simulink model "twelveBalls"  (R2024a)
settings: Solver=FixedStepAuto  StartTime=0.0  StopTime=config.t_max  FixedStep=config.timestep  RelTol=1e-3
undefined symbols (not defined in the file or in its folder): agentsInfo, config, DiscIntNeverNeededParam, Sim3dSensor
libraries: sim3dlib x14, dspvision x1, visionsinks x1
(part 1 of 2)
settings Model: Creator=alexs  LastModifiedBy=alexs

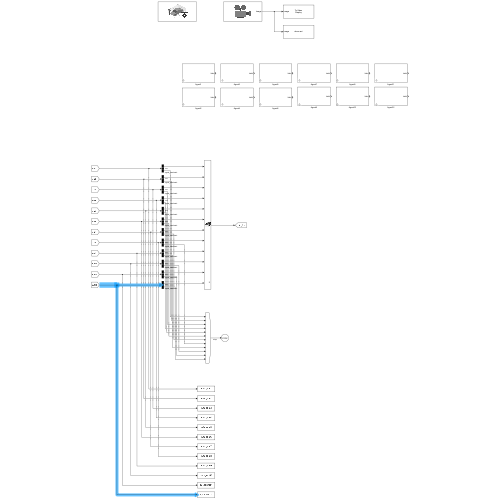
[thumbnail: Simulink's stored preview of the top-level diagram]
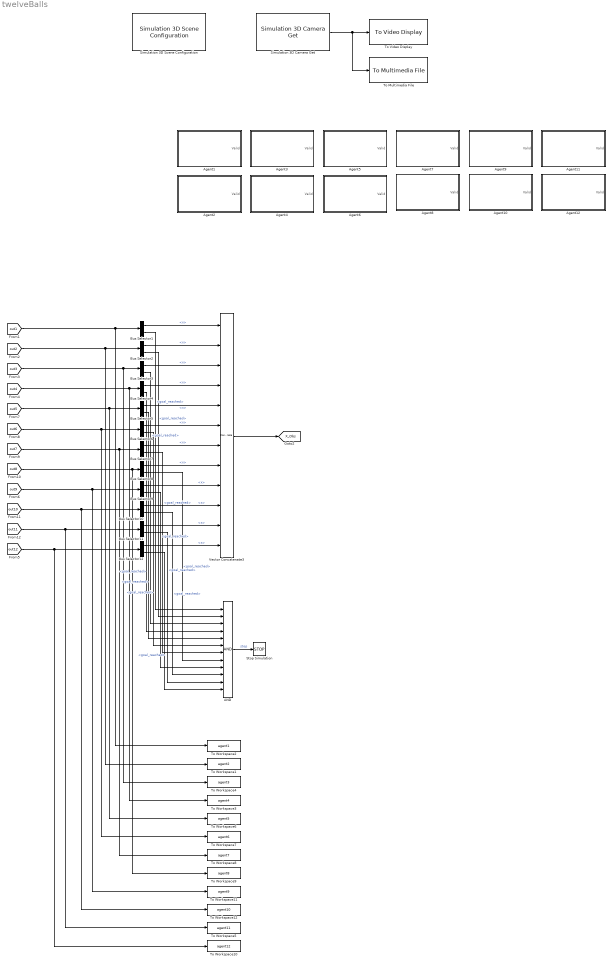
== system twelveBalls ==
  AND : Logic  Inputs=12  IconShape=distinctive  AllPortsSameDT=off  OutDataTypeStr=boolean
  Agent1 : Subsystem  mask{id=1, allAgentsInfo=agentsInfo}
      mask prompts: id "Identifier"; allAgentsInfo "Agents information"
  Agent10 : Subsystem  mask{id=10, allAgentsInfo=agentsInfo}
      mask prompts: id "Identifier"; allAgentsInfo "Agents information"
  Agent11 : Subsystem  mask{id=11, allAgentsInfo=agentsInfo}
      mask prompts: id "Identifier"; allAgentsInfo "Agents information"
  Agent12 : Subsystem  mask{id=12, allAgentsInfo=agentsInfo}
      mask prompts: id "Identifier"; allAgentsInfo "Agents information"
  Agent2 : Subsystem  mask{id=2, allAgentsInfo=agentsInfo}
      mask prompts: id "Identifier"; allAgentsInfo "Agents information"
  Agent3 : Subsystem  mask{id=3, allAgentsInfo=agentsInfo}
      mask prompts: id "Identifier"; allAgentsInfo "Agents information"
  Agent4 : Subsystem  mask{id=4, allAgentsInfo=agentsInfo}
      mask prompts: id "Identifier"; allAgentsInfo "Agents information"
  Agent5 : Subsystem  mask{id=5, allAgentsInfo=agentsInfo}
      mask prompts: id "Identifier"; allAgentsInfo "Agents information"
  Agent6 : Subsystem  mask{id=6, allAgentsInfo=agentsInfo}
      mask prompts: id "Identifier"; allAgentsInfo "Agents information"
  Agent7 : Subsystem  mask{id=7, allAgentsInfo=agentsInfo}
      mask prompts: id "Identifier"; allAgentsInfo "Agents information"
  Agent8 : Subsystem  mask{id=8, allAgentsInfo=agentsInfo}
      mask prompts: id "Identifier"; allAgentsInfo "Agents information"
  Agent9 : Subsystem  mask{id=9, allAgentsInfo=agentsInfo}
      mask prompts: id "Identifier"; allAgentsInfo "Agents information"
  Bus Selector{1..12} (12 alike) : BusSelector  OutputSignals=x,goal_reached
  Simulation 3D Camera Get : sim3dlib/Simulation 3D Camera Get  Priority=1  sensorTag=Sim3dSensor�  sensorId=1  sensorName=Sim3dSensor�  vehTagList={'Scene Origin';'actor1'}  vehTag=Scene Origin  mountLoc=Origin  offsetFlag=on  tmountOffset=cameraTranslation  rmountOffset=cameraRotation  HorizontalResolution=1280  VerticalResolution=720  HorizontalFOV=60  SampleTime=-1  mountPoint=[0 0 20]  mountOrientation=[0 -90 -90]  aMode=5  ID=1
      settings: LibrarySourceBlock=sl3dlib/Simulation 3D/Utilities/Simulation 3D Camera Get
  Simulation 3D Scene Configuration : sim3dlib/Simulation 3D Scene Configuration  Priority=0  ProjectFormat=Default Scenes  SceneDesc=Empty scene  ProjectName=C:\Program Files\MATLAB\R2024a\toolbox\shared\sim3d_projects\automotive_project_windows\UE\WindowsNoEditor\VehicleSimulation.exe  ScenePath=/Game/Maps/HwStrght  EnableOpenDRIVE=off  vehTagList={'Custom';'Scene Origin'}  vehTag=Scene Origin  FreeCameraInitialTranslation=[0, 0, 0]  FreeCameraDefaultInitialTranslation=[-6, 0, 2]  FreeCameraInitialRotation=[0, 0, 0]  FreeCameraDefaultInitialRotation=[0, -15, 0]  OpVisEn=off  Ts=config.timestep  EnableWindow=off  EnableRemoteAccess=off  EnableWeather=off  SunAzimuth=90  SunAltitude=40.0  EnableGeospatialSun=off  Latitude=0  Longitude=0  Date=2023-01-01  Time=10:30:00  GeoTimeZone=-5.0  SunDaylightSaving=off  wind=1  clouds=10  EnableVolumetricClouds=off  CloudCoverage=0  CloudAltitude=6  fog=0  rain=0  RaindropsEffect=off  SnowDensity=0  EnableGeospatial=off  UseTrueOrigin=off  OriginHeight=200  OriginLatitude=40.744652  OriginLongitude=-73.988864  MapStyle=Aerial  AdditionalAssetIDs=[]  UseAdvancedSunSky=off  SolarTime=11  TimeZone=-5  Day=21  Month=9  Year=2022  UseDaylightSavingTime=on  DSTStartDay=10  DSTStartMonth=3  DSTEndDay=3  DSTEndMonth=11  DSTSwitchHour=2  sensorTag=MainCamera1  sensorId=1  sensorName=MainCamera1  mountLoc=Origin  offsetFlag=off  tmountOffset=[0, 0, 0]  rmountOffset=[0, 0, 0]  HorizontalResolution=1280  VerticalResolution=720  HorizontalFOV=60  mountPoint=[0 0 0]  mountOrientation=[0 0 0]  aMode=5  ID=1  GeoTrigger=Inactive
      settings: LibrarySourceBlock=sl3dlib/Simulation 3D/Environment/Simulation 3D Scene Configuration
  Stop Simulation : Stop
  To Multimedia File : dspvision/To Multimedia File  outputFilename=demo.avi  streamSelection=Video only  videoCompressor=None (uncompressed)  audioCompressor=None (uncompressed)  imagePorts=One multidimensional signal  fileType=AVI  audioDatatype=Determine from input data type  fourcc=RGB  audioBitRate=128  audioQuality=75  videoQuality=75  mj2000CompFactor=10
      settings: LibrarySourceBlock=visionsinks/To Multimedia File
  To Video Display : visionsinks/To Video Display  windowSizeMode=Normal  openAtMdlStart=on  fullScreen=off  videoWindowX=678  videoWindowY=374  saveWindowSize=off  videoWindowWidth=1052  videoWindowHeight=706  inputColorFormat=RGB  inputType=Obsolete  imagePorts=One multidimensional signal  OutputDevice=On-screen video monitor  dataOrg=Column-major  isWindowOpen=off
  To Workspace1 : ToWorkspace  VariableName=agent2  SaveFormat=Timeseries  SampleTime=-1
  To Workspace10 : ToWorkspace  VariableName=agent12  SaveFormat=Timeseries  SampleTime=-1
  To Workspace11 : ToWorkspace  VariableName=agent9  SaveFormat=Timeseries  SampleTime=-1
  To Workspace12 : ToWorkspace  VariableName=agent10  SaveFormat=Timeseries  SampleTime=-1
  To Workspace2 : ToWorkspace  VariableName=agent1  SaveFormat=Timeseries  SampleTime=-1
  To Workspace3 : ToWorkspace  VariableName=agent4  SaveFormat=Timeseries  SampleTime=-1
  To Workspace4 : ToWorkspace  VariableName=agent3  SaveFormat=Timeseries  SampleTime=-1
  To Workspace5 : ToWorkspace  VariableName=agent11  SaveFormat=Timeseries  SampleTime=-1
  To Workspace6 : ToWorkspace  VariableName=agent5  SaveFormat=Timeseries  SampleTime=-1
  To Workspace7 : ToWorkspace  VariableName=agent6  SaveFormat=Timeseries  SampleTime=-1
  To Workspace8 : ToWorkspace  VariableName=agent7  SaveFormat=Timeseries  SampleTime=-1
  To Workspace9 : ToWorkspace  VariableName=agent8  SaveFormat=Timeseries  SampleTime=-1
  Vector Concatenate3 : Concatenate  NumInputs=12  Mode=Multidimensional array  ConcatenateDimension=2
  tag scope: X_Obs=global
  wires:
  Simulation 3D Camera Get/1 -> To Multimedia File/1, To Video Display/1
  Bus Selector7/1 -> Vector Concatenate3/7  "<x>"
  Bus Selector3/2 -> AND/3  "<goal_reached>"
  [out1] -> Bus Selector1/1, To Workspace2/1
  Bus Selector1/1 -> Vector Concatenate3/1  "<x>"
  [out7] -> Bus Selector7/1, To Workspace8/1
  [out4] -> Bus Selector4/1, To Workspace3/1
  Bus Selector2/1 -> Vector Concatenate3/2  "<x>"
  Bus Selector8/2 -> AND/8  "<goal_reached>"
  [out2] -> Bus Selector2/1, To Workspace1/1
  Vector Concatenate3/1 -> [X_Obs]
  [out8] -> Bus Selector8/1, To Workspace9/1
  Bus Selector1/2 -> AND/1  "<goal_reached>"
  [out3] -> Bus Selector3/1, To Workspace4/1
  Bus Selector6/2 -> AND/6  "<goal_reached>"
  Bus Selector5/2 -> AND/5  "<goal_reached>"
  Bus Selector2/2 -> AND/2  "<goal_reached>"
  [out6] -> To Workspace7/1, Bus Selector6/1
  Bus Selector4/2 -> AND/4  "<goal_reached>"
  Bus Selector8/1 -> Vector Concatenate3/8  "<x>"
  Bus Selector3/1 -> Vector Concatenate3/3  "<x>"
  Bus Selector4/1 -> Vector Concatenate3/4  "<x>"
  Bus Selector6/1 -> Vector Concatenate3/6  "<x>"
  [out5] -> Bus Selector5/1, To Workspace6/1
  Bus Selector7/2 -> AND/7  "<goal_reached>"
  AND/1 -> Stop Simulation/1  "stop"
  Bus Selector5/1 -> Vector Concatenate3/5  "<x>"
  [out9] -> To Workspace11/1, Bus Selector9/1
  [out10] -> To Workspace12/1, Bus Selector10/1
  [out11] -> To Workspace5/1, Bus Selector11/1
  [out12] -> To Workspace10/1, Bus Selector12/1
  Bus Selector9/1 -> Vector Concatenate3/9  "<x>"
  Bus Selector10/1 -> Vector Concatenate3/10  "<x>"
  Bus Selector11/1 -> Vector Concatenate3/11  "<x>"
  Bus Selector12/1 -> Vector Concatenate3/12  "<x>"
  Bus Selector9/2 -> AND/9  "<goal_reached>"
  Bus Selector10/2 -> AND/10  "<goal_reached>"
  Bus Selector11/2 -> AND/11  "<goal_reached>"
  Bus Selector12/2 -> AND/12  "<goal_reached>"

== system twelveBalls/Agent1 ==
  Actor : Subsystem
  Bus Selector1 : BusSelector  OutputSignals=u
  Controller : Subsystem  mask{id=id, allAgentsInfo=agentsInfo}
      mask prompts: id "Identifier"; allAgentsInfo "Information for all agents"
  Valid : Outport
  tag scope: out1=global
  wires:
  Actor/3(v) -> Controller/2(v)
  Controller/1(out_data) -> Bus Selector1/1, [out1]
  Actor/2(p) -> Controller/1(p)
  Bus Selector1/1 -> Actor/1(u_in)  "<u>"
  [X_Obs] -> Controller/3(X_Obs)
  Actor/1(Valid) -> Valid/1
  Actor/4(overlap_event) -> Controller/4(overlap_event)

== system twelveBalls/Agent10 ==
  Actor : Subsystem
  Bus Selector1 : BusSelector  OutputSignals=u
  Controller : Subsystem  mask{id=id, allAgentsInfo=agentsInfo}
      mask prompts: id "Identifier"; allAgentsInfo "Information for all agents"
  Valid : Outport
  tag scope: out10=global
  wires:
  Actor/3(v) -> Controller/2(v)
  Controller/1(out_data) -> Bus Selector1/1, [out10]
  Actor/2(p) -> Controller/1(p)
  Bus Selector1/1 -> Actor/1(u_in)  "<u>"
  [X_Obs] -> Controller/3(X_Obs)
  Actor/1(Valid) -> Valid/1
  Actor/4(overlap_event) -> Controller/4(overlap_event)

== system twelveBalls/Agent11 ==
  Actor : Subsystem
  Bus Selector1 : BusSelector  OutputSignals=u
  Controller : Subsystem  mask{id=id, allAgentsInfo=agentsInfo}
      mask prompts: id "Identifier"; allAgentsInfo "Information for all agents"
  Valid : Outport
  tag scope: out11=global
  wires:
  Actor/4(overlap_event) -> Controller/4(overlap_event)
  Actor/1(Valid) -> Valid/1
  [X_Obs] -> Controller/3(X_Obs)
  Bus Selector1/1 -> Actor/1(u_in)  "<u>"
  Actor/2(p) -> Controller/1(p)
  Controller/1(out_data) -> [out11], Bus Selector1/1
  Actor/3(v) -> Controller/2(v)

== system twelveBalls/Agent12 ==
  Actor : Subsystem
  Bus Selector1 : BusSelector  OutputSignals=u
  Controller : Subsystem  mask{id=id, allAgentsInfo=agentsInfo}
      mask prompts: id "Identifier"; allAgentsInfo "Information for all agents"
  Valid : Outport
  tag scope: out12=global
  wires:
  Actor/3(v) -> Controller/2(v)
  Controller/1(out_data) -> Bus Selector1/1, [out12]
  Actor/2(p) -> Controller/1(p)
  Bus Selector1/1 -> Actor/1(u_in)  "<u>"
  [X_Obs] -> Controller/3(X_Obs)
  Actor/1(Valid) -> Valid/1
  Actor/4(overlap_event) -> Controller/4(overlap_event)

== system twelveBalls/Agent2 ==
  Actor : Subsystem
  Bus Selector1 : BusSelector  OutputSignals=u
  Controller : Subsystem  mask{id=id, allAgentsInfo=agentsInfo}
      mask prompts: id "Identifier"; allAgentsInfo "Information for all agents"
  Valid : Outport
  tag scope: out2=global
  wires:
  Actor/4(overlap_event) -> Controller/4(overlap_event)
  Actor/1(Valid) -> Valid/1
  [X_Obs] -> Controller/3(X_Obs)
  Bus Selector1/1 -> Actor/1(u_in)  "<u>"
  Actor/2(p) -> Controller/1(p)
  Controller/1(out_data) -> [out2], Bus Selector1/1
  Actor/3(v) -> Controller/2(v)

== system twelveBalls/Agent3 ==
  Actor : Subsystem
  Bus Selector1 : BusSelector  OutputSignals=u
  Controller : Subsystem  mask{id=id, allAgentsInfo=agentsInfo}
      mask prompts: id "Identifier"; allAgentsInfo "Information for all agents"
  Valid : Outport
  tag scope: out3=global
  wires:
  Actor/3(v) -> Controller/2(v)
  Controller/1(out_data) -> Bus Selector1/1, [out3]
  Actor/2(p) -> Controller/1(p)
  Bus Selector1/1 -> Actor/1(u_in)  "<u>"
  [X_Obs] -> Controller/3(X_Obs)
  Actor/1(Valid) -> Valid/1
  Actor/4(overlap_event) -> Controller/4(overlap_event)

== system twelveBalls/Agent4 ==
  Actor : Subsystem
  Bus Selector1 : BusSelector  OutputSignals=u
  Controller : Subsystem  mask{id=id, allAgentsInfo=agentsInfo}
      mask prompts: id "Identifier"; allAgentsInfo "Information for all agents"
  Valid : Outport
  tag scope: out4=global
  wires:
  Actor/4(overlap_event) -> Controller/4(overlap_event)
  Actor/1(Valid) -> Valid/1
  [X_Obs] -> Controller/3(X_Obs)
  Bus Selector1/1 -> Actor/1(u_in)  "<u>"
  Actor/2(p) -> Controller/1(p)
  Controller/1(out_data) -> [out4], Bus Selector1/1
  Actor/3(v) -> Controller/2(v)

== system twelveBalls/Agent5 ==
  Actor : Subsystem
  Bus Selector1 : BusSelector  OutputSignals=u
  Controller : Subsystem  mask{id=id, allAgentsInfo=agentsInfo}
      mask prompts: id "Identifier"; allAgentsInfo "Information for all agents"
  Valid : Outport
  tag scope: out5=global
  wires:
  Actor/4(overlap_event) -> Controller/4(overlap_event)
  Actor/1(Valid) -> Valid/1
  [X_Obs] -> Controller/3(X_Obs)
  Bus Selector1/1 -> Actor/1(u_in)  "<u>"
  Actor/2(p) -> Controller/1(p)
  Controller/1(out_data) -> [out5], Bus Selector1/1
  Actor/3(v) -> Controller/2(v)

== system twelveBalls/Agent6 ==
  Actor : Subsystem
  Bus Selector1 : BusSelector  OutputSignals=u
  Controller : Subsystem  mask{id=id, allAgentsInfo=agentsInfo}
      mask prompts: id "Identifier"; allAgentsInfo "Information for all agents"
  Valid : Outport
  tag scope: out6=global
  wires:
  Actor/3(v) -> Controller/2(v)
  Controller/1(out_data) -> Bus Selector1/1, [out6]
  Actor/2(p) -> Controller/1(p)
  Bus Selector1/1 -> Actor/1(u_in)  "<u>"
  [X_Obs] -> Controller/3(X_Obs)
  Actor/1(Valid) -> Valid/1
  Actor/4(overlap_event) -> Controller/4(overlap_event)

== system twelveBalls/Agent7 ==
  Actor : Subsystem
  Bus Selector1 : BusSelector  OutputSignals=u
  Controller : Subsystem  mask{id=id, allAgentsInfo=agentsInfo}
      mask prompts: id "Identifier"; allAgentsInfo "Information for all agents"
  Valid : Outport
  tag scope: out7=global
  wires:
  Actor/3(v) -> Controller/2(v)
  Controller/1(out_data) -> Bus Selector1/1, [out7]
  Actor/2(p) -> Controller/1(p)
  Bus Selector1/1 -> Actor/1(u_in)  "<u>"
  [X_Obs] -> Controller/3(X_Obs)
  Actor/1(Valid) -> Valid/1
  Actor/4(overlap_event) -> Controller/4(overlap_event)

== system twelveBalls/Agent8 ==
  Actor : Subsystem
  Bus Selector1 : BusSelector  OutputSignals=u
  Controller : Subsystem  mask{id=id, allAgentsInfo=agentsInfo}
      mask prompts: id "Identifier"; allAgentsInfo "Information for all agents"
  Valid : Outport
  tag scope: out8=global
  wires:
  Actor/4(overlap_event) -> Controller/4(overlap_event)
  Actor/1(Valid) -> Valid/1
  [X_Obs] -> Controller/3(X_Obs)
  Bus Selector1/1 -> Actor/1(u_in)  "<u>"
  Actor/2(p) -> Controller/1(p)
  Controller/1(out_data) -> [out8], Bus Selector1/1
  Actor/3(v) -> Controller/2(v)

== system twelveBalls/Agent9 ==
  Actor : Subsystem
  Bus Selector1 : BusSelector  OutputSignals=u
  Controller : Subsystem  mask{id=id, allAgentsInfo=agentsInfo}
      mask prompts: id "Identifier"; allAgentsInfo "Information for all agents"
  Valid : Outport
  tag scope: out9=global
  wires:
  Actor/4(overlap_event) -> Controller/4(overlap_event)
  Actor/1(Valid) -> Valid/1
  [X_Obs] -> Controller/3(X_Obs)
  Bus Selector1/1 -> Actor/1(u_in)  "<u>"
  Actor/2(p) -> Controller/1(p)
  Controller/1(out_data) -> [out9], Bus Selector1/1
  Actor/3(v) -> Controller/2(v)

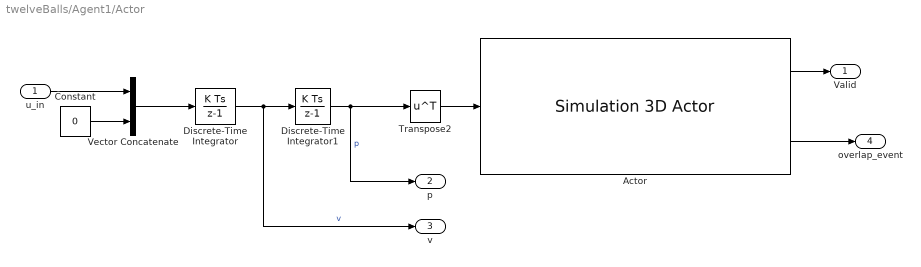
== system twelveBalls/Agent1/Actor ==
  u_in : Inport
  Actor : sim3dlib/Simulation 3D Actor  Priority=1  ActorName=actor1  ParentName=Scene Origin  Operation=Create at setup  InitScriptText=|  SampleTime=-1  Translation=agentsInfo{id}.p'  Rotation=single([0 0 0])  Scale=single([1 1 1])  InputsText=actor1.Translation  EventsText=actor1.BeginOverlapEvent  aMode=5  ActorTag=actor1  ActorType=Sim3dActor  ID=C
      | % Reserved keywords:
      | % - Actor : handle to this actor object
      | % - World : handle to the world object
      | 
      | % Examples:
      | 
      | % Create a primitive geometry (optional)
      | 
      | % Actor.createShape('sphere', [allAgentsInfo{id}.shape(1) allAgentsInfo{id}.shape(2) 1]);
      | 
      | 
      | % Initialize values (optional)
      | % Actor.Scale = 1;
      | % Actor.Gravity = false;
      | % Actor.Physics = true;
      | % Actor.Color = [0 0 1];
      | % Actor.Shininess = 0;
      | % Actor.Mobility = sim3d.utils.MobilityTypes.Movable;
      | % Actor.Shadows = false;
  Constant : Constant  Value=0
  Discrete-Time Integrator : DiscreteIntegrator  InitialCondition=agentsInfo{id}.v  SampleTime=-1  LimitOutput=on  UpperSaturationLimit=config.v_max/sqrt(2)  LowerSaturationLimit=-config.v_max/sqrt(2)  ICPrevOutput=DiscIntNeverNeededParam  ICPrevScaledInput=DiscIntNeverNeededParam
  Discrete-Time Integrator1 : DiscreteIntegrator  InitialCondition=agentsInfo{id}.p  SampleTime=-1  ICPrevOutput=DiscIntNeverNeededParam  ICPrevScaledInput=DiscIntNeverNeededParam
  Transpose2 : Math  Operator=transpose
  Vector Concatenate : Concatenate
  Valid : Outport
  p : Outport  Port=2
  v : Outport  Port=3
  overlap_event : Outport  Port=4
  wires:
  Actor/1 -> Valid/1
  Discrete-Time Integrator1/1 -> Transpose2/1, p/1  "p"
  Discrete-Time Integrator/1 -> Discrete-Time Integrator1/1, v/1  "v"
  Transpose2/1 -> Actor/1
  u_in/1 -> Vector Concatenate/1
  Constant/1 -> Vector Concatenate/2
  Vector Concatenate/1 -> Discrete-Time Integrator/1
  Actor/2 -> overlap_event/1

== system twelveBalls/Agent1/Controller ==
  p : Inport
  v : Inport  Port=2
  X_Obs : Inport  Port=3
  overlap_event : Inport  Port=4
  Bus Creator : BusCreator  Inputs=6
  Clock1 : Clock
  Stop Simulation : Stop
  Vector Concatenate2 : Concatenate
  h_cbf : MATLABSystem  System=h_cbf_system  id=id  config=config  agents_info=agentsInfo  SimulateUsing=Interpreted execution
      mask Type: h_cbf_system
      mask Display:
      | disp('h_cbf_system');
      | port_label('input',1,'t');
      | port_label('input',2,'x');
      | port_label('input',3,'X_obs');
      | port_label('output',1,'u');
      | port_label('output',2,'goal_reached');
      | port_label('output',3,'cost');
      | port_label('output',4,'exit_flag');
  out_data : Outport
  wires:
  Vector Concatenate2/1 -> h_cbf/2, Bus Creator/5  "x"
  h_cbf/4 -> Stop Simulation/1, Bus Creator/4  "exit_flag"
  Bus Creator/1 -> out_data/1
  Clock1/1 -> h_cbf/1
  h_cbf/3 -> Bus Creator/3  "cost"
  p/1 -> Vector Concatenate2/1
  h_cbf/1 -> Bus Creator/1  "u"
  v/1 -> Vector Concatenate2/2
  X_Obs/1 -> h_cbf/3
  h_cbf/2 -> Bus Creator/2  "goal_reached"
  overlap_event/1 -> Bus Creator/6  "overlap_event"

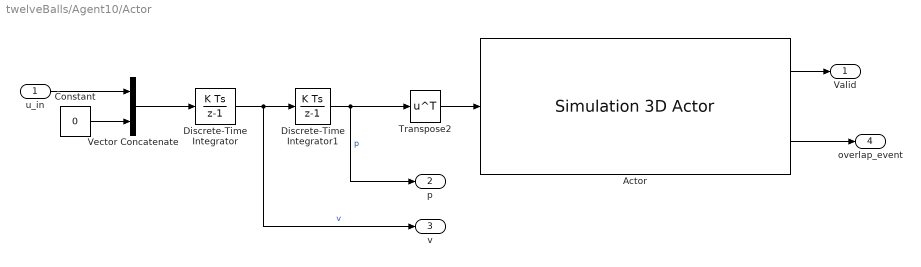
== system twelveBalls/Agent10/Actor ==
  u_in : Inport
  Actor : sim3dlib/Simulation 3D Actor  Priority=1  ActorName=actor10  ParentName=Scene Origin  Operation=Create at setup  InitScriptText=|  SampleTime=-1  Translation=agentsInfo{id}.p'  Rotation=single([0 0 0])  Scale=single([1 1 1])  InputsText=actor10.Translation  EventsText=actor10.BeginOverlapEvent  aMode=5  ActorTag=actor10  ActorType=Sim3dActor  ID=C
      | % Reserved keywords:
      | % - Actor : handle to this actor object
      | % - World : handle to the world object
      | 
      | % Examples:
      | 
      | % Create a primitive geometry (optional)
      | 
      | % Actor.createShape('sphere', [allAgentsInfo{id}.shape(1) allAgentsInfo{id}.shape(2) 1]);
      | 
      | 
      | % Initialize values (optional)
      | % Actor.Scale = 1;
      | % Actor.Gravity = false;
      | % Actor.Physics = true;
      | % Actor.Color = [0 0 1];
      | % Actor.Shininess = 0;
      | % Actor.Mobility = sim3d.utils.MobilityTypes.Movable;
      | % Actor.Shadows = false;
  Constant : Constant  Value=0
  Discrete-Time Integrator : DiscreteIntegrator  InitialCondition=agentsInfo{id}.v  SampleTime=-1  LimitOutput=on  UpperSaturationLimit=config.v_max/sqrt(2)  LowerSaturationLimit=-config.v_max/sqrt(2)  ICPrevOutput=DiscIntNeverNeededParam  ICPrevScaledInput=DiscIntNeverNeededParam
  Discrete-Time Integrator1 : DiscreteIntegrator  InitialCondition=agentsInfo{id}.p  SampleTime=-1  ICPrevOutput=DiscIntNeverNeededParam  ICPrevScaledInput=DiscIntNeverNeededParam
  Transpose2 : Math  Operator=transpose
  Vector Concatenate : Concatenate
  Valid : Outport
  p : Outport  Port=2
  v : Outport  Port=3
  overlap_event : Outport  Port=4
  wires:
  Actor/1 -> Valid/1
  Discrete-Time Integrator1/1 -> Transpose2/1, p/1  "p"
  Discrete-Time Integrator/1 -> Discrete-Time Integrator1/1, v/1  "v"
  Transpose2/1 -> Actor/1
  u_in/1 -> Vector Concatenate/1
  Constant/1 -> Vector Concatenate/2
  Vector Concatenate/1 -> Discrete-Time Integrator/1
  Actor/2 -> overlap_event/1

== system twelveBalls/Agent10/Controller ==
  p : Inport
  v : Inport  Port=2
  X_Obs : Inport  Port=3
  overlap_event : Inport  Port=4
  Bus Creator : BusCreator  Inputs=6
  Clock1 : Clock
  Stop Simulation : Stop
  Vector Concatenate2 : Concatenate
  h_cbf : MATLABSystem  System=h_cbf_system  id=id  config=config  agents_info=agentsInfo  SimulateUsing=Interpreted execution
      mask Type: h_cbf_system
      mask Display:
      | disp('h_cbf_system');
      | port_label('input',1,'t');
      | port_label('input',2,'x');
      | port_label('input',3,'X_obs');
      | port_label('output',1,'u');
      | port_label('output',2,'goal_reached');
      | port_label('output',3,'cost');
      | port_label('output',4,'exit_flag');
  out_data : Outport
  wires:
  Vector Concatenate2/1 -> h_cbf/2, Bus Creator/5  "x"
  h_cbf/4 -> Stop Simulation/1, Bus Creator/4  "exit_flag"
  Bus Creator/1 -> out_data/1
  Clock1/1 -> h_cbf/1
  h_cbf/3 -> Bus Creator/3  "cost"
  p/1 -> Vector Concatenate2/1
  h_cbf/1 -> Bus Creator/1  "u"
  v/1 -> Vector Concatenate2/2
  X_Obs/1 -> h_cbf/3
  h_cbf/2 -> Bus Creator/2  "goal_reached"
  overlap_event/1 -> Bus Creator/6  "overlap_event"

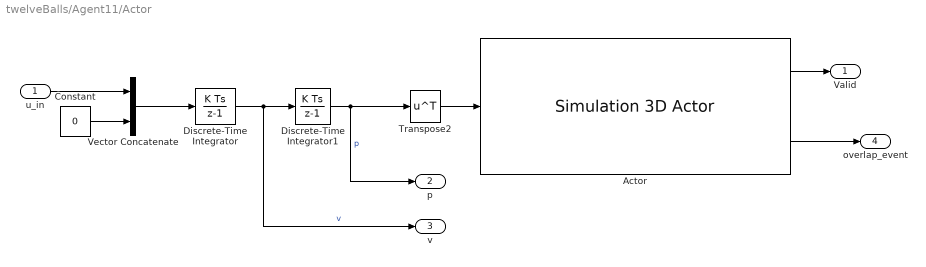
== system twelveBalls/Agent11/Actor ==
  u_in : Inport
  Actor : sim3dlib/Simulation 3D Actor  Priority=1  ActorName=actor11  ParentName=Scene Origin  Operation=Create at setup  InitScriptText=|  SampleTime=-1  Translation=agentsInfo{id}.p'  Rotation=single([0 0 0])  Scale=single([1 1 1])  InputsText=actor11.Translation  EventsText=actor11.BeginOverlapEvent  aMode=5  ActorTag=actor11  ActorType=Sim3dActor  ID=C
      | % Reserved keywords:
      | % - Actor : handle to this actor object
      | % - World : handle to the world object
      | 
      | % Examples:
      | 
      | % Create a primitive geometry (optional)
      | 
      | % Actor.createShape('sphere', [allAgentsInfo{id}.shape(1) allAgentsInfo{id}.shape(2) 1]);
      | 
      | 
      | % Initialize values (optional)
      | % Actor.Scale = 1;
      | % Actor.Gravity = false;
      | % Actor.Physics = true;
      | % Actor.Color = [0 0 1];
      | % Actor.Shininess = 0;
      | % Actor.Mobility = sim3d.utils.MobilityTypes.Movable;
      | % Actor.Shadows = false;
  Constant : Constant  Value=0
  Discrete-Time Integrator : DiscreteIntegrator  InitialCondition=agentsInfo{id}.v  SampleTime=-1  LimitOutput=on  UpperSaturationLimit=config.v_max/sqrt(2)  LowerSaturationLimit=-config.v_max/sqrt(2)  ICPrevOutput=DiscIntNeverNeededParam  ICPrevScaledInput=DiscIntNeverNeededParam
  Discrete-Time Integrator1 : DiscreteIntegrator  InitialCondition=agentsInfo{id}.p  SampleTime=-1  ICPrevOutput=DiscIntNeverNeededParam  ICPrevScaledInput=DiscIntNeverNeededParam
  Transpose2 : Math  Operator=transpose
  Vector Concatenate : Concatenate
  Valid : Outport
  p : Outport  Port=2
  v : Outport  Port=3
  overlap_event : Outport  Port=4
  wires:
  Actor/2 -> overlap_event/1
  Vector Concatenate/1 -> Discrete-Time Integrator/1
  Constant/1 -> Vector Concatenate/2
  u_in/1 -> Vector Concatenate/1
  Transpose2/1 -> Actor/1
  Discrete-Time Integrator/1 -> v/1, Discrete-Time Integrator1/1  "v"
  Discrete-Time Integrator1/1 -> p/1, Transpose2/1  "p"
  Actor/1 -> Valid/1

== system twelveBalls/Agent11/Controller ==
  p : Inport
  v : Inport  Port=2
  X_Obs : Inport  Port=3
  overlap_event : Inport  Port=4
  Bus Creator : BusCreator  Inputs=6
  Clock1 : Clock
  Stop Simulation : Stop
  Vector Concatenate2 : Concatenate
  h_cbf : MATLABSystem  System=h_cbf_system  id=id  config=config  agents_info=agentsInfo  SimulateUsing=Interpreted execution
      mask Type: h_cbf_system
      mask Display:
      | disp('h_cbf_system');
      | port_label('input',1,'t');
      | port_label('input',2,'x');
      | port_label('input',3,'X_obs');
      | port_label('output',1,'u');
      | port_label('output',2,'goal_reached');
      | port_label('output',3,'cost');
      | port_label('output',4,'exit_flag');
  out_data : Outport
  wires:
  overlap_event/1 -> Bus Creator/6  "overlap_event"
  h_cbf/2 -> Bus Creator/2  "goal_reached"
  X_Obs/1 -> h_cbf/3
  v/1 -> Vector Concatenate2/2
  h_cbf/1 -> Bus Creator/1  "u"
  p/1 -> Vector Concatenate2/1
  h_cbf/3 -> Bus Creator/3  "cost"
  Clock1/1 -> h_cbf/1
  Bus Creator/1 -> out_data/1
  h_cbf/4 -> Bus Creator/4, Stop Simulation/1  "exit_flag"
  Vector Concatenate2/1 -> Bus Creator/5, h_cbf/2  "x"

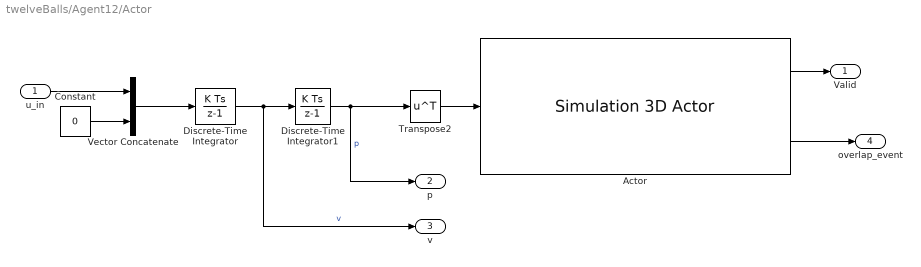
== system twelveBalls/Agent12/Actor ==
  u_in : Inport
  Actor : sim3dlib/Simulation 3D Actor  Priority=1  ActorName=actor12  ParentName=Scene Origin  Operation=Create at setup  InitScriptText=|  SampleTime=-1  Translation=agentsInfo{id}.p'  Rotation=single([0 0 0])  Scale=single([1 1 1])  InputsText=actor12.Translation  EventsText=actor12.BeginOverlapEvent  aMode=5  ActorTag=actor12  ActorType=Sim3dActor  ID=C
      | % Reserved keywords:
      | % - Actor : handle to this actor object
      | % - World : handle to the world object
      | 
      | % Examples:
      | 
      | % Create a primitive geometry (optional)
      | 
      | % Actor.createShape('sphere', [allAgentsInfo{id}.shape(1) allAgentsInfo{id}.shape(2) 1]);
      | 
      | 
      | % Initialize values (optional)
      | % Actor.Scale = 1;
      | % Actor.Gravity = false;
      | % Actor.Physics = true;
      | % Actor.Color = [0 0 1];
      | % Actor.Shininess = 0;
      | % Actor.Mobility = sim3d.utils.MobilityTypes.Movable;
      | % Actor.Shadows = false;
  Constant : Constant  Value=0
  Discrete-Time Integrator : DiscreteIntegrator  InitialCondition=agentsInfo{id}.v  SampleTime=-1  LimitOutput=on  UpperSaturationLimit=config.v_max/sqrt(2)  LowerSaturationLimit=-config.v_max/sqrt(2)  ICPrevOutput=DiscIntNeverNeededParam  ICPrevScaledInput=DiscIntNeverNeededParam
  Discrete-Time Integrator1 : DiscreteIntegrator  InitialCondition=agentsInfo{id}.p  SampleTime=-1  ICPrevOutput=DiscIntNeverNeededParam  ICPrevScaledInput=DiscIntNeverNeededParam
  Transpose2 : Math  Operator=transpose
  Vector Concatenate : Concatenate
  Valid : Outport
  p : Outport  Port=2
  v : Outport  Port=3
  overlap_event : Outport  Port=4
  wires:
  Actor/1 -> Valid/1
  Discrete-Time Integrator1/1 -> Transpose2/1, p/1  "p"
  Discrete-Time Integrator/1 -> Discrete-Time Integrator1/1, v/1  "v"
  Transpose2/1 -> Actor/1
  u_in/1 -> Vector Concatenate/1
  Constant/1 -> Vector Concatenate/2
  Vector Concatenate/1 -> Discrete-Time Integrator/1
  Actor/2 -> overlap_event/1

== system twelveBalls/Agent12/Controller ==
  p : Inport
  v : Inport  Port=2
  X_Obs : Inport  Port=3
  overlap_event : Inport  Port=4
  Bus Creator : BusCreator  Inputs=6
  Clock1 : Clock
  Stop Simulation : Stop
  Vector Concatenate2 : Concatenate
  h_cbf : MATLABSystem  System=h_cbf_system  id=id  config=config  agents_info=agentsInfo  SimulateUsing=Interpreted execution
      mask Type: h_cbf_system
      mask Display:
      | disp('h_cbf_system');
      | port_label('input',1,'t');
      | port_label('input',2,'x');
      | port_label('input',3,'X_obs');
      | port_label('output',1,'u');
      | port_label('output',2,'goal_reached');
      | port_label('output',3,'cost');
      | port_label('output',4,'exit_flag');
  out_data : Outport
  wires:
  Vector Concatenate2/1 -> h_cbf/2, Bus Creator/5  "x"
  h_cbf/4 -> Stop Simulation/1, Bus Creator/4  "exit_flag"
  Bus Creator/1 -> out_data/1
  Clock1/1 -> h_cbf/1
  h_cbf/3 -> Bus Creator/3  "cost"
  p/1 -> Vector Concatenate2/1
  h_cbf/1 -> Bus Creator/1  "u"
  v/1 -> Vector Concatenate2/2
  X_Obs/1 -> h_cbf/3
  h_cbf/2 -> Bus Creator/2  "goal_reached"
  overlap_event/1 -> Bus Creator/6  "overlap_event"

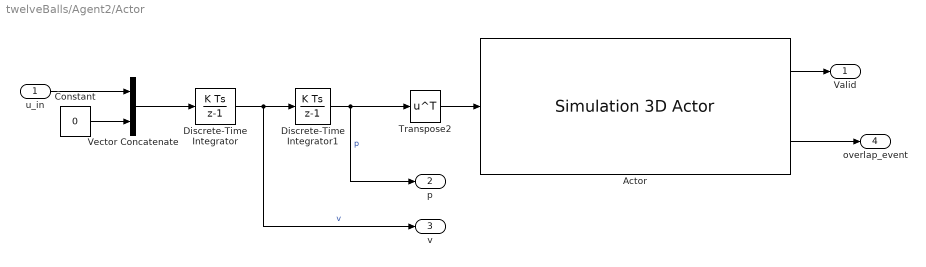
== system twelveBalls/Agent2/Actor ==
  u_in : Inport
  Actor : sim3dlib/Simulation 3D Actor  Priority=1  ActorName=actor2  ParentName=Scene Origin  Operation=Create at setup  InitScriptText=|  SampleTime=-1  Translation=agentsInfo{id}.p'  Rotation=single([0 0 0])  Scale=single([1 1 1])  InputsText=actor2.Translation  EventsText=actor2.BeginOverlapEvent  aMode=5  ActorTag=actor2  ActorType=Sim3dActor  ID=C
      | % Reserved keywords:
      | % - Actor : handle to this actor object
      | % - World : handle to the world object
      | 
      | % Examples:
      | 
      | % Create a primitive geometry (optional)
      | 
      | % Actor.createShape('sphere', [allAgentsInfo{id}.shape(1) allAgentsInfo{id}.shape(2) 1]);
      | 
      | 
      | % Initialize values (optional)
      | % Actor.Scale = 1;
      | % Actor.Gravity = false;
      | % Actor.Physics = true;
      | % Actor.Color = [0 0 1];
      | % Actor.Shininess = 0;
      | % Actor.Mobility = sim3d.utils.MobilityTypes.Movable;
      | % Actor.Shadows = false;
  Constant : Constant  Value=0
  Discrete-Time Integrator : DiscreteIntegrator  InitialCondition=agentsInfo{id}.v  SampleTime=-1  LimitOutput=on  UpperSaturationLimit=config.v_max/sqrt(2)  LowerSaturationLimit=-config.v_max/sqrt(2)  ICPrevOutput=DiscIntNeverNeededParam  ICPrevScaledInput=DiscIntNeverNeededParam
  Discrete-Time Integrator1 : DiscreteIntegrator  InitialCondition=agentsInfo{id}.p  SampleTime=-1  ICPrevOutput=DiscIntNeverNeededParam  ICPrevScaledInput=DiscIntNeverNeededParam
  Transpose2 : Math  Operator=transpose
  Vector Concatenate : Concatenate
  Valid : Outport
  p : Outport  Port=2
  v : Outport  Port=3
  overlap_event : Outport  Port=4
  wires:
  Actor/2 -> overlap_event/1
  Vector Concatenate/1 -> Discrete-Time Integrator/1
  Constant/1 -> Vector Concatenate/2
  u_in/1 -> Vector Concatenate/1
  Transpose2/1 -> Actor/1
  Discrete-Time Integrator/1 -> v/1, Discrete-Time Integrator1/1  "v"
  Discrete-Time Integrator1/1 -> p/1, Transpose2/1  "p"
  Actor/1 -> Valid/1

== system twelveBalls/Agent2/Controller ==
  p : Inport
  v : Inport  Port=2
  X_Obs : Inport  Port=3
  overlap_event : Inport  Port=4
  Bus Creator : BusCreator  Inputs=6
  Clock1 : Clock
  Stop Simulation : Stop
  Vector Concatenate2 : Concatenate
  h_cbf : MATLABSystem  System=h_cbf_system  id=id  config=config  agents_info=agentsInfo  SimulateUsing=Interpreted execution
      mask Type: h_cbf_system
      mask Display:
      | disp('h_cbf_system');
      | port_label('input',1,'t');
      | port_label('input',2,'x');
      | port_label('input',3,'X_obs');
      | port_label('output',1,'u');
      | port_label('output',2,'goal_reached');
      | port_label('output',3,'cost');
      | port_label('output',4,'exit_flag');
  out_data : Outport
  wires:
  overlap_event/1 -> Bus Creator/6  "overlap_event"
  h_cbf/2 -> Bus Creator/2  "goal_reached"
  X_Obs/1 -> h_cbf/3
  v/1 -> Vector Concatenate2/2
  h_cbf/1 -> Bus Creator/1  "u"
  p/1 -> Vector Concatenate2/1
  h_cbf/3 -> Bus Creator/3  "cost"
  Clock1/1 -> h_cbf/1
  Bus Creator/1 -> out_data/1
  h_cbf/4 -> Bus Creator/4, Stop Simulation/1  "exit_flag"
  Vector Concatenate2/1 -> Bus Creator/5, h_cbf/2  "x"

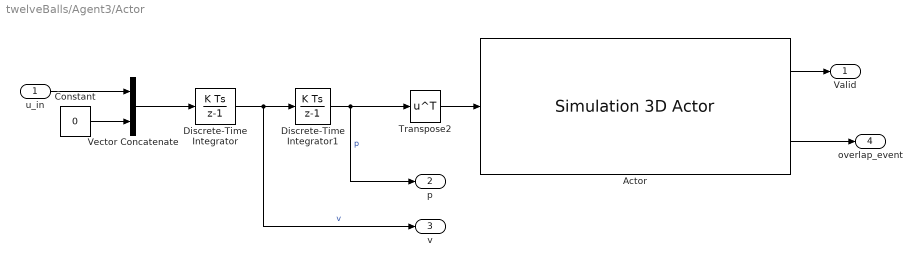
== system twelveBalls/Agent3/Actor ==
  u_in : Inport
  Actor : sim3dlib/Simulation 3D Actor  Priority=1  ActorName=actor3  ParentName=Scene Origin  Operation=Create at setup  InitScriptText=|  SampleTime=-1  Translation=agentsInfo{id}.p'  Rotation=single([0 0 0])  Scale=single([1 1 1])  InputsText=actor3.Translation  EventsText=actor3.BeginOverlapEvent  aMode=5  ActorTag=actor3  ActorType=Sim3dActor  ID=C
      | % Reserved keywords:
      | % - Actor : handle to this actor object
      | % - World : handle to the world object
      | 
      | % Examples:
      | 
      | % Create a primitive geometry (optional)
      | 
      | % Actor.createShape('sphere', [allAgentsInfo{id}.shape(1) allAgentsInfo{id}.shape(2) 1]);
      | 
      | 
      | % Initialize values (optional)
      | % Actor.Scale = 1;
      | % Actor.Gravity = false;
      | % Actor.Physics = true;
      | % Actor.Color = [0 0 1];
      | % Actor.Shininess = 0;
      | % Actor.Mobility = sim3d.utils.MobilityTypes.Movable;
      | % Actor.Shadows = false;
  Constant : Constant  Value=0
  Discrete-Time Integrator : DiscreteIntegrator  InitialCondition=agentsInfo{id}.v  SampleTime=-1  LimitOutput=on  UpperSaturationLimit=config.v_max/sqrt(2)  LowerSaturationLimit=-config.v_max/sqrt(2)  ICPrevOutput=DiscIntNeverNeededParam  ICPrevScaledInput=DiscIntNeverNeededParam
  Discrete-Time Integrator1 : DiscreteIntegrator  InitialCondition=agentsInfo{id}.p  SampleTime=-1  ICPrevOutput=DiscIntNeverNeededParam  ICPrevScaledInput=DiscIntNeverNeededParam
  Transpose2 : Math  Operator=transpose
  Vector Concatenate : Concatenate
  Valid : Outport
  p : Outport  Port=2
  v : Outport  Port=3
  overlap_event : Outport  Port=4
  wires:
  Actor/1 -> Valid/1
  Discrete-Time Integrator1/1 -> Transpose2/1, p/1  "p"
  Discrete-Time Integrator/1 -> Discrete-Time Integrator1/1, v/1  "v"
  Transpose2/1 -> Actor/1
  u_in/1 -> Vector Concatenate/1
  Constant/1 -> Vector Concatenate/2
  Vector Concatenate/1 -> Discrete-Time Integrator/1
  Actor/2 -> overlap_event/1

== system twelveBalls/Agent3/Controller ==
  p : Inport
  v : Inport  Port=2
  X_Obs : Inport  Port=3
  overlap_event : Inport  Port=4
  Bus Creator : BusCreator  Inputs=6
  Clock1 : Clock
  Stop Simulation : Stop
  Vector Concatenate2 : Concatenate
  h_cbf : MATLABSystem  System=h_cbf_system  id=id  config=config  agents_info=agentsInfo  SimulateUsing=Interpreted execution
      mask Type: h_cbf_system
      mask Display:
      | disp('h_cbf_system');
      | port_label('input',1,'t');
      | port_label('input',2,'x');
      | port_label('input',3,'X_obs');
      | port_label('output',1,'u');
      | port_label('output',2,'goal_reached');
      | port_label('output',3,'cost');
      | port_label('output',4,'exit_flag');
  out_data : Outport
  wires:
  Vector Concatenate2/1 -> h_cbf/2, Bus Creator/5  "x"
  h_cbf/4 -> Stop Simulation/1, Bus Creator/4  "exit_flag"
  Bus Creator/1 -> out_data/1
  Clock1/1 -> h_cbf/1
  h_cbf/3 -> Bus Creator/3  "cost"
  p/1 -> Vector Concatenate2/1
  h_cbf/1 -> Bus Creator/1  "u"
  v/1 -> Vector Concatenate2/2
  X_Obs/1 -> h_cbf/3
  h_cbf/2 -> Bus Creator/2  "goal_reached"
  overlap_event/1 -> Bus Creator/6  "overlap_event"

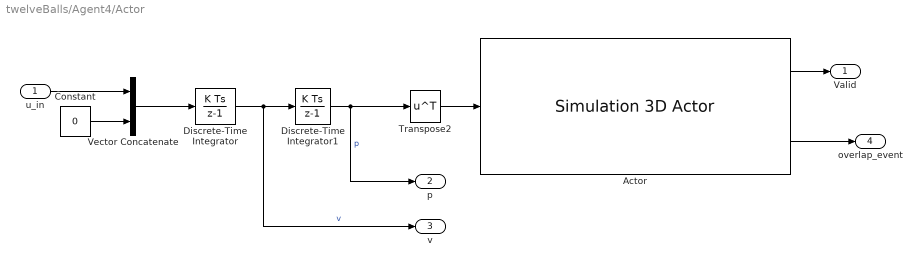
== system twelveBalls/Agent4/Actor ==
  u_in : Inport
  Actor : sim3dlib/Simulation 3D Actor  Priority=1  ActorName=actor4  ParentName=Scene Origin  Operation=Create at setup  InitScriptText=|  SampleTime=-1  Translation=agentsInfo{id}.p'  Rotation=single([0 0 0])  Scale=single([1 1 1])  InputsText=actor4.Translation  EventsText=actor4.BeginOverlapEvent  aMode=5  ActorTag=actor4  ActorType=Sim3dActor  ID=C
      | % Reserved keywords:
      | % - Actor : handle to this actor object
      | % - World : handle to the world object
      | 
      | % Examples:
      | 
      | % Create a primitive geometry (optional)
      | 
      | % Actor.createShape('sphere', [allAgentsInfo{id}.shape(1) allAgentsInfo{id}.shape(2) 1]);
      | 
      | 
      | % Initialize values (optional)
      | % Actor.Scale = 1;
      | % Actor.Gravity = false;
      | % Actor.Physics = true;
      | % Actor.Color = [0 0 1];
      | % Actor.Shininess = 0;
      | % Actor.Mobility = sim3d.utils.MobilityTypes.Movable;
      | % Actor.Shadows = false;
  Constant : Constant  Value=0
  Discrete-Time Integrator : DiscreteIntegrator  InitialCondition=agentsInfo{id}.v  SampleTime=-1  LimitOutput=on  UpperSaturationLimit=config.v_max/sqrt(2)  LowerSaturationLimit=-config.v_max/sqrt(2)  ICPrevOutput=DiscIntNeverNeededParam  ICPrevScaledInput=DiscIntNeverNeededParam
  Discrete-Time Integrator1 : DiscreteIntegrator  InitialCondition=agentsInfo{id}.p  SampleTime=-1  ICPrevOutput=DiscIntNeverNeededParam  ICPrevScaledInput=DiscIntNeverNeededParam
  Transpose2 : Math  Operator=transpose
  Vector Concatenate : Concatenate
  Valid : Outport
  p : Outport  Port=2
  v : Outport  Port=3
  overlap_event : Outport  Port=4
  wires:
  Actor/2 -> overlap_event/1
  Vector Concatenate/1 -> Discrete-Time Integrator/1
  Constant/1 -> Vector Concatenate/2
  u_in/1 -> Vector Concatenate/1
  Transpose2/1 -> Actor/1
  Discrete-Time Integrator/1 -> v/1, Discrete-Time Integrator1/1  "v"
  Discrete-Time Integrator1/1 -> p/1, Transpose2/1  "p"
  Actor/1 -> Valid/1

== system twelveBalls/Agent4/Controller ==
  p : Inport
  v : Inport  Port=2
  X_Obs : Inport  Port=3
  overlap_event : Inport  Port=4
  Bus Creator : BusCreator  Inputs=6
  Clock1 : Clock
  Stop Simulation : Stop
  Vector Concatenate2 : Concatenate
  h_cbf : MATLABSystem  System=h_cbf_system  id=id  config=config  agents_info=agentsInfo  SimulateUsing=Interpreted execution
      mask Type: h_cbf_system
      mask Display:
      | disp('h_cbf_system');
      | port_label('input',1,'t');
      | port_label('input',2,'x');
      | port_label('input',3,'X_obs');
      | port_label('output',1,'u');
      | port_label('output',2,'goal_reached');
      | port_label('output',3,'cost');
      | port_label('output',4,'exit_flag');
  out_data : Outport
  wires:
  overlap_event/1 -> Bus Creator/6  "overlap_event"
  h_cbf/2 -> Bus Creator/2  "goal_reached"
  X_Obs/1 -> h_cbf/3
  v/1 -> Vector Concatenate2/2
  h_cbf/1 -> Bus Creator/1  "u"
  p/1 -> Vector Concatenate2/1
  h_cbf/3 -> Bus Creator/3  "cost"
  Clock1/1 -> h_cbf/1
  Bus Creator/1 -> out_data/1
  h_cbf/4 -> Bus Creator/4, Stop Simulation/1  "exit_flag"
  Vector Concatenate2/1 -> Bus Creator/5, h_cbf/2  "x"

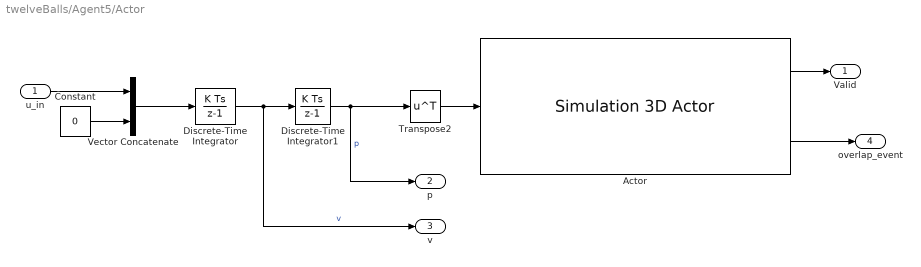
== system twelveBalls/Agent5/Actor ==
  u_in : Inport
  Actor : sim3dlib/Simulation 3D Actor  Priority=1  ActorName=actor5  ParentName=Scene Origin  Operation=Create at setup  InitScriptText=|  SampleTime=-1  Translation=agentsInfo{id}.p'  Rotation=single([0 0 0])  Scale=single([1 1 1])  InputsText=actor5.Translation  EventsText=actor5.BeginOverlapEvent  aMode=5  ActorTag=actor5  ActorType=Sim3dActor  ID=C
      | % Reserved keywords:
      | % - Actor : handle to this actor object
      | % - World : handle to the world object
      | 
      | % Examples:
      | 
      | % Create a primitive geometry (optional)
      | 
      | % Actor.createShape('sphere', [allAgentsInfo{id}.shape(1) allAgentsInfo{id}.shape(2) 1]);
      | 
      | 
      | % Initialize values (optional)
      | % Actor.Scale = 1;
      | % Actor.Gravity = false;
      | % Actor.Physics = true;
      | % Actor.Color = [0 0 1];
      | % Actor.Shininess = 0;
      | % Actor.Mobility = sim3d.utils.MobilityTypes.Movable;
      | % Actor.Shadows = false;
  Constant : Constant  Value=0
  Discrete-Time Integrator : DiscreteIntegrator  InitialCondition=agentsInfo{id}.v  SampleTime=-1  LimitOutput=on  UpperSaturationLimit=config.v_max/sqrt(2)  LowerSaturationLimit=-config.v_max/sqrt(2)  ICPrevOutput=DiscIntNeverNeededParam  ICPrevScaledInput=DiscIntNeverNeededParam
  Discrete-Time Integrator1 : DiscreteIntegrator  InitialCondition=agentsInfo{id}.p  SampleTime=-1  ICPrevOutput=DiscIntNeverNeededParam  ICPrevScaledInput=DiscIntNeverNeededParam
  Transpose2 : Math  Operator=transpose
  Vector Concatenate : Concatenate
  Valid : Outport
  p : Outport  Port=2
  v : Outport  Port=3
  overlap_event : Outport  Port=4
  wires:
  Actor/2 -> overlap_event/1
  Vector Concatenate/1 -> Discrete-Time Integrator/1
  Constant/1 -> Vector Concatenate/2
  u_in/1 -> Vector Concatenate/1
  Transpose2/1 -> Actor/1
  Discrete-Time Integrator/1 -> v/1, Discrete-Time Integrator1/1  "v"
  Discrete-Time Integrator1/1 -> p/1, Transpose2/1  "p"
  Actor/1 -> Valid/1

== system twelveBalls/Agent5/Controller ==
  p : Inport
  v : Inport  Port=2
  X_Obs : Inport  Port=3
  overlap_event : Inport  Port=4
  Bus Creator : BusCreator  Inputs=6
  Clock1 : Clock
  Stop Simulation : Stop
  Vector Concatenate2 : Concatenate
  h_cbf : MATLABSystem  System=h_cbf_system  id=id  config=config  agents_info=agentsInfo  SimulateUsing=Interpreted execution
      mask Type: h_cbf_system
      mask Display:
      | disp('h_cbf_system');
      | port_label('input',1,'t');
      | port_label('input',2,'x');
      | port_label('input',3,'X_obs');
      | port_label('output',1,'u');
      | port_label('output',2,'goal_reached');
      | port_label('output',3,'cost');
      | port_label('output',4,'exit_flag');
  out_data : Outport
  wires:
  overlap_event/1 -> Bus Creator/6  "overlap_event"
  h_cbf/2 -> Bus Creator/2  "goal_reached"
  X_Obs/1 -> h_cbf/3
  v/1 -> Vector Concatenate2/2
  h_cbf/1 -> Bus Creator/1  "u"
  p/1 -> Vector Concatenate2/1
  h_cbf/3 -> Bus Creator/3  "cost"
  Clock1/1 -> h_cbf/1
  Bus Creator/1 -> out_data/1
  h_cbf/4 -> Bus Creator/4, Stop Simulation/1  "exit_flag"
  Vector Concatenate2/1 -> Bus Creator/5, h_cbf/2  "x"

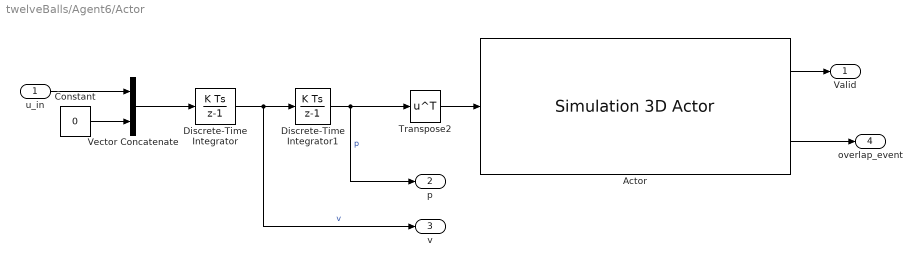
== system twelveBalls/Agent6/Actor ==
  u_in : Inport
  Actor : sim3dlib/Simulation 3D Actor  Priority=1  ActorName=actor6  ParentName=Scene Origin  Operation=Create at setup  InitScriptText=|  SampleTime=-1  Translation=agentsInfo{id}.p'  Rotation=single([0 0 0])  Scale=single([1 1 1])  InputsText=actor6.Translation  EventsText=actor6.BeginOverlapEvent  aMode=5  ActorTag=actor6  ActorType=Sim3dActor  ID=C
      | % Reserved keywords:
      | % - Actor : handle to this actor object
      | % - World : handle to the world object
      | 
      | % Examples:
      | 
      | % Create a primitive geometry (optional)
      | 
      | % Actor.createShape('sphere', [allAgentsInfo{id}.shape(1) allAgentsInfo{id}.shape(2) 1]);
      | 
      | 
      | % Initialize values (optional)
      | % Actor.Scale = 1;
      | % Actor.Gravity = false;
      | % Actor.Physics = true;
      | % Actor.Color = [0 0 1];
      | % Actor.Shininess = 0;
      | % Actor.Mobility = sim3d.utils.MobilityTypes.Movable;
      | % Actor.Shadows = false;
  Constant : Constant  Value=0
  Discrete-Time Integrator : DiscreteIntegrator  InitialCondition=agentsInfo{id}.v  SampleTime=-1  LimitOutput=on  UpperSaturationLimit=config.v_max/sqrt(2)  LowerSaturationLimit=-config.v_max/sqrt(2)  ICPrevOutput=DiscIntNeverNeededParam  ICPrevScaledInput=DiscIntNeverNeededParam
  Discrete-Time Integrator1 : DiscreteIntegrator  InitialCondition=agentsInfo{id}.p  SampleTime=-1  ICPrevOutput=DiscIntNeverNeededParam  ICPrevScaledInput=DiscIntNeverNeededParam
  Transpose2 : Math  Operator=transpose
  Vector Concatenate : Concatenate
  Valid : Outport
  p : Outport  Port=2
  v : Outport  Port=3
  overlap_event : Outport  Port=4
  wires:
  Actor/1 -> Valid/1
  Discrete-Time Integrator1/1 -> Transpose2/1, p/1  "p"
  Discrete-Time Integrator/1 -> Discrete-Time Integrator1/1, v/1  "v"
  Transpose2/1 -> Actor/1
  u_in/1 -> Vector Concatenate/1
  Constant/1 -> Vector Concatenate/2
  Vector Concatenate/1 -> Discrete-Time Integrator/1
  Actor/2 -> overlap_event/1

== system twelveBalls/Agent6/Controller ==
  p : Inport
  v : Inport  Port=2
  X_Obs : Inport  Port=3
  overlap_event : Inport  Port=4
  Bus Creator : BusCreator  Inputs=6
  Clock1 : Clock
  Stop Simulation : Stop
  Vector Concatenate2 : Concatenate
  h_cbf : MATLABSystem  System=h_cbf_system  id=id  config=config  agents_info=agentsInfo  SimulateUsing=Interpreted execution
      mask Type: h_cbf_system
      mask Display:
      | disp('h_cbf_system');
      | port_label('input',1,'t');
      | port_label('input',2,'x');
      | port_label('input',3,'X_obs');
      | port_label('output',1,'u');
      | port_label('output',2,'goal_reached');
      | port_label('output',3,'cost');
      | port_label('output',4,'exit_flag');
  out_data : Outport
  wires:
  Vector Concatenate2/1 -> h_cbf/2, Bus Creator/5  "x"
  h_cbf/4 -> Stop Simulation/1, Bus Creator/4  "exit_flag"
  Bus Creator/1 -> out_data/1
  Clock1/1 -> h_cbf/1
  h_cbf/3 -> Bus Creator/3  "cost"
  p/1 -> Vector Concatenate2/1
  h_cbf/1 -> Bus Creator/1  "u"
  v/1 -> Vector Concatenate2/2
  X_Obs/1 -> h_cbf/3
  h_cbf/2 -> Bus Creator/2  "goal_reached"
  overlap_event/1 -> Bus Creator/6  "overlap_event"

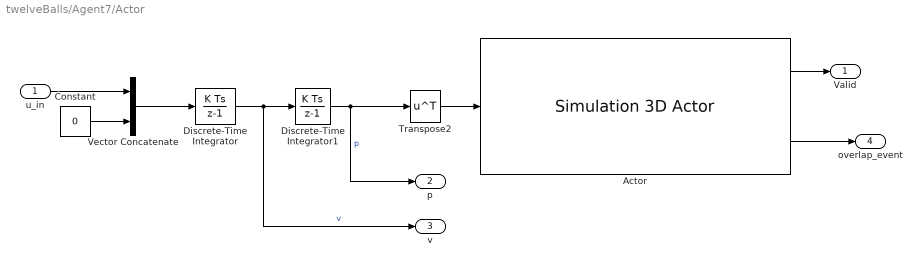
== system twelveBalls/Agent7/Actor ==
  u_in : Inport
  Actor : sim3dlib/Simulation 3D Actor  Priority=1  ActorName=actor7  ParentName=Scene Origin  Operation=Create at setup  InitScriptText=|  SampleTime=-1  Translation=agentsInfo{id}.p'  Rotation=single([0 0 0])  Scale=single([1 1 1])  InputsText=actor7.Translation  EventsText=actor7.BeginOverlapEvent  aMode=5  ActorTag=actor7  ActorType=Sim3dActor  ID=C
      | % Reserved keywords:
      | % - Actor : handle to this actor object
      | % - World : handle to the world object
      | 
      | % Examples:
      | 
      | % Create a primitive geometry (optional)
      | 
      | % Actor.createShape('sphere', [allAgentsInfo{id}.shape(1) allAgentsInfo{id}.shape(2) 1]);
      | 
      | 
      | % Initialize values (optional)
      | % Actor.Scale = 1;
      | % Actor.Gravity = false;
      | % Actor.Physics = true;
      | % Actor.Color = [0 0 1];
      | % Actor.Shininess = 0;
      | % Actor.Mobility = sim3d.utils.MobilityTypes.Movable;
      | % Actor.Shadows = false;
  Constant : Constant  Value=0
  Discrete-Time Integrator : DiscreteIntegrator  InitialCondition=agentsInfo{id}.v  SampleTime=-1  LimitOutput=on  UpperSaturationLimit=config.v_max/sqrt(2)  LowerSaturationLimit=-config.v_max/sqrt(2)  ICPrevOutput=DiscIntNeverNeededParam  ICPrevScaledInput=DiscIntNeverNeededParam
  Discrete-Time Integrator1 : DiscreteIntegrator  InitialCondition=agentsInfo{id}.p  SampleTime=-1  ICPrevOutput=DiscIntNeverNeededParam  ICPrevScaledInput=DiscIntNeverNeededParam
  Transpose2 : Math  Operator=transpose
  Vector Concatenate : Concatenate
  Valid : Outport
  p : Outport  Port=2
  v : Outport  Port=3
  overlap_event : Outport  Port=4
  wires:
  Actor/1 -> Valid/1
  Discrete-Time Integrator1/1 -> Transpose2/1, p/1  "p"
  Discrete-Time Integrator/1 -> Discrete-Time Integrator1/1, v/1  "v"
  Transpose2/1 -> Actor/1
  u_in/1 -> Vector Concatenate/1
  Constant/1 -> Vector Concatenate/2
  Vector Concatenate/1 -> Discrete-Time Integrator/1
  Actor/2 -> overlap_event/1

== system twelveBalls/Agent7/Controller ==
  p : Inport
  v : Inport  Port=2
  X_Obs : Inport  Port=3
  overlap_event : Inport  Port=4
  Bus Creator : BusCreator  Inputs=6
  Clock1 : Clock
  Stop Simulation : Stop
  Vector Concatenate2 : Concatenate
  h_cbf : MATLABSystem  System=h_cbf_system  id=id  config=config  agents_info=agentsInfo  SimulateUsing=Interpreted execution
      mask Type: h_cbf_system
      mask Display:
      | disp('h_cbf_system');
      | port_label('input',1,'t');
      | port_label('input',2,'x');
      | port_label('input',3,'X_obs');
      | port_label('output',1,'u');
      | port_label('output',2,'goal_reached');
      | port_label('output',3,'cost');
      | port_label('output',4,'exit_flag');
  out_data : Outport
  wires:
  Vector Concatenate2/1 -> h_cbf/2, Bus Creator/5  "x"
  h_cbf/4 -> Stop Simulation/1, Bus Creator/4  "exit_flag"
  Bus Creator/1 -> out_data/1
  Clock1/1 -> h_cbf/1
  h_cbf/3 -> Bus Creator/3  "cost"
  p/1 -> Vector Concatenate2/1
  h_cbf/1 -> Bus Creator/1  "u"
  v/1 -> Vector Concatenate2/2
  X_Obs/1 -> h_cbf/3
  h_cbf/2 -> Bus Creator/2  "goal_reached"
  overlap_event/1 -> Bus Creator/6  "overlap_event"

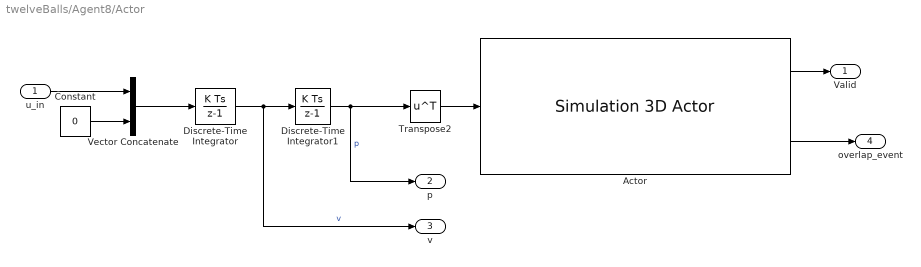
== system twelveBalls/Agent8/Actor ==
  u_in : Inport
  Actor : sim3dlib/Simulation 3D Actor  Priority=1  ActorName=actor8  ParentName=Scene Origin  Operation=Create at setup  InitScriptText=|  SampleTime=-1  Translation=agentsInfo{id}.p'  Rotation=single([0 0 0])  Scale=single([1 1 1])  InputsText=actor8.Translation  EventsText=actor8.BeginOverlapEvent  aMode=5  ActorTag=actor8  ActorType=Sim3dActor  ID=C
      | % Reserved keywords:
      | % - Actor : handle to this actor object
      | % - World : handle to the world object
      | 
      | % Examples:
      | 
      | % Create a primitive geometry (optional)
      | 
      | % Actor.createShape('sphere', [allAgentsInfo{id}.shape(1) allAgentsInfo{id}.shape(2) 1]);
      | 
      | 
      | % Initialize values (optional)
      | % Actor.Scale = 1;
      | % Actor.Gravity = false;
      | % Actor.Physics = true;
      | % Actor.Color = [0 0 1];
      | % Actor.Shininess = 0;
      | % Actor.Mobility = sim3d.utils.MobilityTypes.Movable;
      | % Actor.Shadows = false;
  Constant : Constant  Value=0
  Discrete-Time Integrator : DiscreteIntegrator  InitialCondition=agentsInfo{id}.v  SampleTime=-1  LimitOutput=on  UpperSaturationLimit=config.v_max/sqrt(2)  LowerSaturationLimit=-config.v_max/sqrt(2)  ICPrevOutput=DiscIntNeverNeededParam  ICPrevScaledInput=DiscIntNeverNeededParam
  Discrete-Time Integrator1 : DiscreteIntegrator  InitialCondition=agentsInfo{id}.p  SampleTime=-1  ICPrevOutput=DiscIntNeverNeededParam  ICPrevScaledInput=DiscIntNeverNeededParam
  Transpose2 : Math  Operator=transpose
  Vector Concatenate : Concatenate
  Valid : Outport
  p : Outport  Port=2
  v : Outport  Port=3
  overlap_event : Outport  Port=4
  wires:
  Actor/2 -> overlap_event/1
  Vector Concatenate/1 -> Discrete-Time Integrator/1
  Constant/1 -> Vector Concatenate/2
  u_in/1 -> Vector Concatenate/1
  Transpose2/1 -> Actor/1
  Discrete-Time Integrator/1 -> v/1, Discrete-Time Integrator1/1  "v"
  Discrete-Time Integrator1/1 -> p/1, Transpose2/1  "p"
  Actor/1 -> Valid/1
